simulink model "Inyectora_DigitalTwin"  (R2026b)
settings: Solver=VariableStepAuto  StopTime=inf  AbsTol=1e-3  EnableMultiTasking=on
values from neighbouring files (symbols this model uses):
  t_apertura = 2.0    (= 2)    [init_params.m]
  t_cierre = 2.0    (= 2)    [init_params.m]
  t_enfriamiento = 10.0    (= 10)    [init_params.m]
  t_inyeccion = 3.0    (= 3)    [init_params.m]
  t_mantenimiento = 4.0    (= 4)    [init_params.m]
libraries: simulink x1
settings Model: Creator=Rogue  LastModifiedBy=Rogue
settings SolverCC: AutoScaleAbsTol=off
settings DataIOCC: LimitDataPoints=on  MaxDataPoints=10000
settings OptimizationCC: LifeSpan=inf  ReuseModelBlockBuffer=off
settings DebuggingCC: AllowSymbolicDim=off  ArithmeticOperatorsInVariantConditions=warning  SFExecutionAtInitializationDiag=none  SFNoUnconditionalDefaultTransitionDiag=warning  SFUnexpectedBacktrackingDiag=warning  SubsystemReferenceDiagnosticForUnitTest=warning
settings SFSimCC: CustomCodeUndefinedFunction=UseInterfaceOnly  SimUseLocalCustomCode=off
settings RTWCC: DLArmComputeVersion=19.05  RTWUseLocalCustomCode=off
settings CodeAppCC: StateflowObjectComments=on
settings GRTTargetCC: TargetLangStandard=C89/C90 (ANSI)
settings ConfigComp: CovExternalEMLEnable=off  CovSFcnEnable=off  CovSaveCumulativeToWorkspaceVar=on  CovSaveSingleToWorkspaceVar=on
settings SimscapeCC: SimscapeLogType=all  SimscapeUseEnergyAccounting=off
settings ExplorerConfigSet: InternalSimMechanicsExplorerSettings=|
  | <ExplorerConfiguration>
  | 
  |   <canonicalview>default</canonicalview>
  | 
  |   <TilePanel>
  |     <TileInfo>
  |       <Tiles Columns="1" Count="1" Height="610" Rows="1" Width="1078">
  |         <Row Weight="1"/>
  |         <Column Weight="1"/>
  |         <Tile Height="1" Width="1" X="0" Y="0"/>
  |       </Tiles>
  |     </TileInfo>
  |     <SceneInfo>
  |       <SceneViewer>
  |         <IsThisViewStd>
  |           <IsStandardView>off</IsStandardView>
  |           <StandardViewName>Front</StandardViewName>
  |         </IsThisViewStd>
  |         <BGColor>
  |           <R>1</R>
  |           <G>1</G>
  |           <B>1</B>
  |           <A>1</A>
  |         </BGColor>
  |         <Camera>
  |           <DoPerspective>off</DoPerspective>
  |           <Position>
  |             <X>-4.8151858056067729</X>
  |             <Y>-0.45425897153882505</Y>
  |             <Z>-0.29583074117817348</Z>
  |           </Position>
  |           <Center>
  |             <X>0.3283322810866165</X>
  |             <Y>0.1741945047826792</Y>
  |             <Z>0.090521326187803119</Z>
  |           </Center>
  |           <Up>
  |             <X>0.075415500852524311</X>
  |             <Y>-0.89165566740071944</Y>
  |             <Z>0.4463884777000191</Z>
  |           </Up>
  |           <XLim>0.93528457740457382</XLim>
  |           <YLim>0.93528457740457382</YLim>
  |           <ViewLimDist>0.01</ViewLimDist>
  |         </Camera>
  |       </SceneViewer>
  |     </SceneInfo>
  |   </TilePanel>
  | 
  |   <MechEditorPanel>
  |     <GfxPanelCameraMap/>
  |     <Cameras/>
  |     <VideoCreator>
  |       <IncludeTiles>All</IncludeTiles>
  |       <IncludeTime>on</IncludeTime>
  |       <IncludeWorldFrame>off</IncludeWorldFrame>
  |       <PlaybackSpeedRatio>1</PlaybackSpeedRatio>
  |       <FrameRate>30</FrameRate>
  |       <FrameSize>auto</FrameSize>
  |       <VideoFormat>UncompressedAVI</VideoFormat>
  |     </VideoCreator>
  |   </MechEditorPanel>
  | 
  |   <PlaybackSettings>
  |     <PlaybackSpeedFactor>4</PlaybackSpeedFactor>
  |   </PlaybackSettings>
  | 
  | </ExplorerConfiguration>

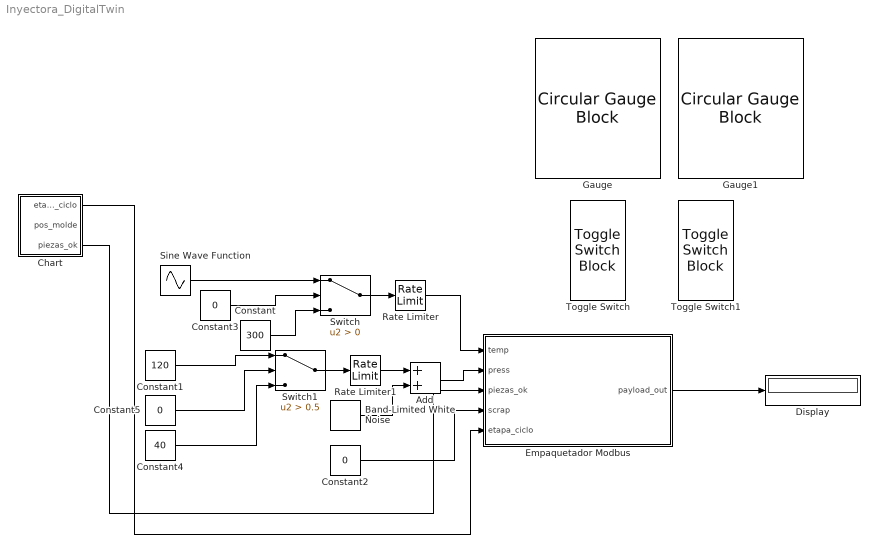
== system Inyectora_DigitalTwin ==
  Add : Sum
  Band-Limited White Noise : simulink/Sources/Band-Limited White Noise  Cov=[0.1]  Ts=0.1  seed=[23341]
  Chart : Stateflow chart  TreatAsAtomicUnit=on
  Constant : Constant  Value=300
  Constant1 : Constant  Value=120
  Constant2 : Constant  Value=0
  Constant3 : Constant  Value=0
  Constant4 : Constant  Value=40
  Constant5 : Constant  Value=0
  Display : Display
  Empaquetador Modbus : MATLAB Function  TreatAsAtomicUnit=on
  Gauge : CircularGaugeBlock  LabelPosition=Bottom  ScaleMax=300  FontColor=[0.0, 0.0, 0.0]
  Gauge1 : CircularGaugeBlock  LabelPosition=Bottom  ScaleMax=200  FontColor=[0.0, 0.0, 0.0]
  Rate Limiter : RateLimiter  RisingSlewLimit=2  FallingSlewLimit=-5  SampleTimeMode=inherited
  Rate Limiter1 : RateLimiter  RisingSlewLimit=20  FallingSlewLimit=-20  SampleTimeMode=inherited
  Sine Wave Function : Sin  TimeSource=Use external signal  Bias=259  SampleTime=0
  Switch : Switch  Criteria=u2 > Threshold  SaturateOnIntegerOverflow=off  InputSameDT=off
  Switch1 : Switch  Criteria=u2 > Threshold  Threshold=0.5  SaturateOnIntegerOverflow=off  InputSameDT=off
  Toggle Switch : ToggleSwitchBlock
  Toggle Switch1 : ToggleSwitchBlock
  wires:
  Chart/1(etapa_ciclo) -> Empaquetador Modbus/5(etapa_ciclo)
  Constant2/1 -> Empaquetador Modbus/4(scrap)
  Chart/3(piezas_ok) -> Empaquetador Modbus/3(piezas_ok)
  Empaquetador Modbus/1(payload_out) -> Display/1
  Sine Wave Function/1 -> Switch/1
  Constant3/1 -> Switch/2
  Switch/1 -> Rate Limiter/1
  Rate Limiter/1 -> Empaquetador Modbus/1(temp)
  Constant/1 -> Switch/3
  Constant1/1 -> Switch1/1
  Constant4/1 -> Switch1/3
  Constant5/1 -> Switch1/2
  Switch1/1 -> Rate Limiter1/1
  Rate Limiter1/1 -> Add/1
  Band-Limited White Noise/1 -> Add/2
  Add/1 -> Empaquetador Modbus/2(press)

== matlab function Inyectora_DigitalTwin/Empaquetador Modbus ==
  data: temp input; payload_out output; press input; piezas_ok input; scrap input; etapa_ciclo input
function payload_out = empaquetar_udp(temp, press, piezas_ok, scrap, etapa_ciclo)
% 1. Inicializar array de 9 elementos uint16 (18 bytes)
payload_out = zeros(1, 9, 'uint16');

% 2. Mapeo de datos fijos
payload_out(1) = uint16(1); % Máquina ID = 1 (En el otro archivo pon 2)
payload_out(2) = uint16(etapa_ciclo);

% 3. LÓGICA DE FALLAS
falla = 0; % Estado normal
if temp > 275
    falla = 1; % Falla Térmica
elseif press < 80
    falla = 2; % Falla Presión
end

% Asignar el código de falla a la posición 3
payload_out(3) = uint16(falla);

% 4. Producción
payload_out(4) = uint16(piezas_ok);
payload_out(5) = uint16(scrap);

% 5. Convertir Float32 a 2x uint16 (Temp y Presión)
temp_bytes = typecast(single(temp), 'uint16');
payload_out(6) = temp_bytes(1);
payload_out(7) = temp_bytes(2);

press_bytes = typecast(single(press), 'uint16');
payload_out(8) = press_bytes(1);
payload_out(9) = press_bytes(2);

% 6. Enviar a NestJS
enviar_udp(payload_out);
end

== stateflow chart Inyectora_DigitalTwin/Chart ==
  state CERRANDO
    etapa_ciclo = 1; pos_molde = 0.4
  state ABRIENDO
    etapa_ciclo = 5; pos_molde = 0;
    piezas_ok = piezas_ok + 1;
  state INYECTANDO
    etapa_ciclo = 2; pos_molde = 0.4
  state ENFRIANDO
    etapa_ciclo = 4; pos_molde = 0.4
  state MANTENIMIENTO
    etapa_ciclo = 3; pos_molde = 0.4;
  (default) -> CERRANDO
  ABRIENDO -> CERRANDO : after(t_apertura, sec)
  CERRANDO -> INYECTANDO : after(t_cierre, sec)
  ENFRIANDO -> ABRIENDO : after(t_enfriamiento, sec)
  INYECTANDO -> MANTENIMIENTO : after(t_inyeccion, sec)
  MANTENIMIENTO -> ENFRIANDO : after(t_mantenimiento, sec)
  data: etapa_ciclo output; pos_molde output; t_apertura parameter; t_cierre parameter; t_enfriamiento parameter; t_inyeccion parameter; t_mantenimiento parameter; piezas_ok output double size=1 =0
